simulink model "UIT"  (R2022b)
settings: Solver=VariableStepAuto  StartTime=0.0  StopTime=1e4  RelTol=1e-3
settings Model: Creator=lenovo  LastModifiedBy=lenovo

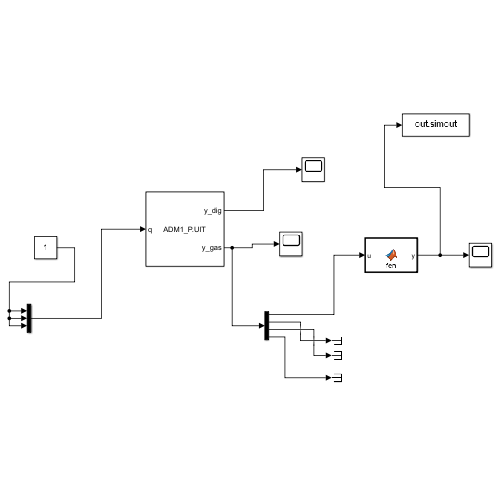
[thumbnail: Simulink's stored preview of the top-level diagram]
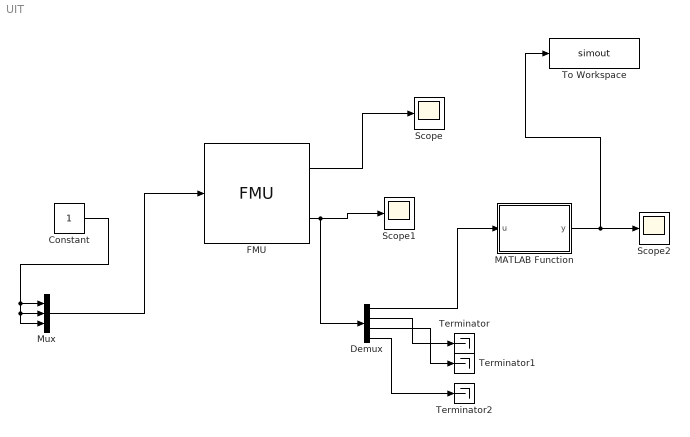
== system UIT ==
  Constant : Constant
  Demux : Demux
  FMU : FMU  FMUName=ADM1_P_UIT.fmu  FMUMode=ModelExchange  Gas_Meter=struct('D_ch4',1.57E-9,'D_co2',1.98E-9,'D_h2',4.65E-9,'D_n2',1.7777777777777777E-9,'D_nh3',1.9560185185185183E-9,'D_o2',2.8E-9,'P_atm',1.013,'T0',298.15,'T_op_mean',315.15,'T_ref_k',308.15,'V_gas',100.0,'V_liq',3400.0,'kla',200.0)  P_block_jacobian_check=off  P_block_jacobian_check_tol=1.0E-6  P_block_solver_experimental_mode=int32(0)  P_block_solver_profiling=off  P_cs_experimental_mode=int32(0)  P_cs_profiling=off  P_cs_rel_tol=1.0E-6  P_cs_solver=int32(0)  P_cs_step_size=0.001  P_enforce_bounds=on  P_events_default_tol=1.0E-10  P_events_tol_factor=1.0E-4  P_iteration_variable_scaling=int32(1)  P_log_level=int32(3)  P_log_start_time=-1.0E20  P_log_stop_time=1.0E20  P_mathematical_domain_warnings_limit=int32(-1)  P_nle_active_bounds_mode=int32(0)  P_nle_brent_ignore_error=off  P_nle_jacobian_calculation_mode=int32(0)  P_nle_jacobian_finite_difference_delta=1.490116119384766E-8  P_nle_jacobian_update_mode=int32(2)  P_nle_solver_check_jac_cond=off  P_nle_solver_default_tol=1.0E-10  P_nle_solver_exit_criterion=int32(3)  P_nle_solver_max_iter=int32(100)  P_nle_solver_max_iter_no_jacobian=int32(10)  P_nle_solver_max_residual_scaling_factor=1.0E10  P_nle_solver_min_residual_scaling_factor=1.0E-10  P_nle_solver_min_tol=1.0E-12  P_nle_solver_regularization_tolerance=-1.0  P_nle_solver_step_limit_factor=10.0  P_nle_solver_tol_factor=1.0E-4  P_nle_solver_use_last_integrator_step=on  P_nle_solver_use_nominals_as_fallback=on  P_rescale_after_singular_jac=on  P_rescale_each_step=off  P_residual_equation_scaling=int32(1)  P_runtime_log_to_file=off  P_time_events_default_tol=2.220446049250313E-14  P_use_Brent_in_1d=on  P_use_jacobian_equilibration=off  P_use_newton_for_brent=on  combiTimeTable=struct('columns',[int32(2),int32(3),int32(4),int32(5),int32(6),int32(7),int32(8),int32(9),int32(10),int32(11),int32(12),int32(13),int32(14),int32(15),int32(16),int32(17),int32(18),int32(19),int32(20),int32(21),int32(22),int32(23),int32(24),int32(25),int32(26),int32(27)],'offset',[0.0],'startTime',0.0,'table',reshape([0.0,1.0,2.0,0.0,1.0,4.0], [3,2]),'timeEvents',int32(1),'verboseRead',boolean(true))  combiTimeTable_fileName=C:/Users/lenovo/Desktop/KINGSTON/DOTTORATO/Modelica/Pilot_plant/Codig_Ari_Aprile 2023/txt_new/sAntonio_CattleSlurry_nir.txt  combiTimeTable_tableName=Input_CattleSlurry  combiTimeTable1=struct('columns',[int32(2),int32(3),int32(4),int32(5),int32(6),int32(7),int32(8),int32(9),int32(10),int32(11),int32(12),int32(13),int32(14),int32(15),int32(16),int32(17),int32(18),int32(19),int32(20),int32(21),int32(22),int32(23),int32(24),int32(25),int32(26),int32(27)],'offset',[0.0],'startTime',0.0,'table',reshape([0.0,1.0,2.0,0.0,1.0,4.0], [3,2]),'timeEvents',int32(1),'verboseRead',boolean(true))  combiTimeTable1_fileName=C:/Users/lenovo/Desktop/KINGSTON/DOTTORATO/Modelica/Pilot_plant/Codig_Ari_Aprile 2023/txt_new/sAntonio_MaizeSilage_nir.txt  combiTimeTable1_tableName=Input_MaizeSilage  combiTimeTable2=struct('columns',[int32(2),int32(3),int32(4),int32(5),int32(6),int32(7),int32(8),int32(9),int32(10),int32(11),int32(12),int32(13),int32(14),int32(15),int32(16),int32(17),int32(18),int32(19),int32(20),int32(21),int32(22),int32(23),int32(24),int32(25),int32(26),int32(27)],'offset',[0.0],'startTime',0.0,'table',reshape([0.0,1.0,2.0,0.0,1.0,4.0], [3,2]),'timeEvents',int32(1),'verboseRead',boolean(true))  combiTimeTable2_fileName=C:/Users/lenovo/Desktop/KINGSTON/DOTTORATO/Modelica/Pilot_plant/Codig_Ari_Aprile 2023/txt_new/UIT_TomatoSouce_nir.txt  combiTimeTable2_tableName=Input_TomatoSouce  combiTimeTable3=struct('columns',[int32(2),int32(3),int32(4),int32(5),int32(6),int32(7),int32(8),int32(9),int32(10),int32(11),int32(12),int32(13),int32(14),int32(15),int32(16),int32(17),int32(18),int32(19),int32(20),int32(21),int32(22),int32(23),int32(24),int32(25),int32(26),int32(27)],'offset',[0.0],'startTime',0.0,'table',reshape([0.0,1.0,2.0,0.0,1.0,4.0], [3,2]),'timeEvents',int32(1),'verboseRead',boolean(true))  combiTimeTable3_fileName=C:/Users/lenovo/Desktop/KINGSTON/DOTTORATO/Modelica/Pilot_plant/Codig_Ari_Aprile 2023/txt_new/sAntonio_TomatoPeels_nir.txt  combiTimeTable3_tableName=Input_TomatoPeels  combiTimeTable4=struct('columns',[int32(2)],'offset',[0.0],'startTime',0.0,'table',reshape([0.0,150.0,240.0,2000.0,0.0,37.0,0.0,37.0], [4,2]),'timeEvents',int32(1),'verboseRead',boolean(true))  combiTimeTable4_fileName=NoName  combiTimeTable4_tableName=NoName  combiTimeTable5=struct('columns',[int32(2)],'offset',[0.0],'startTime',0.0,'table',reshape([0.0,150.0,240.0,2000.0,37.0,0.0,37.0,37.0], [4,2]),'timeEvents',int32(1),'verboseRead',boolean(true))  combiTimeTable5_fileName=NoName  combiTimeTable5_tableName=NoName  digester=struct('COD_VS_PR_BCA',1.58,'D_ch4',1.57E-9,'D_co2',1.98E-9,'D_h2',4.65E-9,'D_n2',1.7777777777777777E-9,'D_nh3',1.9560185185185183E-9,'D_o2',2.8E-9,'Ki_h2_c4',1.0E-5,'Ki_h2_fa',5.0E-6,'Ki_h2_pro',3.5E-6,'Ki_nh3_ac',0.0018,'Ks_IN',1.0E-4,'Ks_IP',2.0E-5,'Ks_aa',0.3,'Ks_ac',0.15,'Ks_c4',0.1,'Ks_fa',0.4,'Ks_h2',2.5E-5,'Ks_pro',0.3,'Ks_su',0.5,'N_PR',7.5,'P_atm',1.013,'S_aa_start',0.0260061,'S_ac_start',0.259353,'S_an_start',0.0156,'S_bu_start',0.00643617,'S_ca_start',3.28398E-5,'S_cat_start',0.121528,'S_ch4_start',0.277401,'S_fa_start',0.0444521,'S_gas_ch4_start',1.27265,'S_gas_co2_start',0.0164995,'S_gas_h2_start',5.30538E-6,'S_gas_nh3_start',3.35695E-6,'S_h2_start',6.87765E-7,'S_i_start',0.193985,'S_ic_start',0.255202,'S_in_start',0.157029,'S_ip_start',0.00496694,'S_mg_start',5.62229E-5,'S_pro_start',0.050891,'S_su_start',0.0246664,'S_va_start',0.00353521,'T0',298.15,'T_op_mean',315.15,'T_ref',298.15,'T_ref_k',308.15,'Tref_khyd',[308.15,308.15,308.15,308.15,308.15,308.15,308.15,308.15],'V_gas',0.0172,'V_liq',0.012,'X_aa_start',0.566877,'X_ac_start',1.32145,'X_acp_start',8.78817E-12,'X_c4_start',0.498118,'X_c_start',0.0,'X_ccm_start',0.00543116,'X_ch_start',[0.82044,0.712461,10.3487],'X_fa_start',0.288931,'X_h2_start',0.621273,'X_i_start',36.0924,'X_li_start',0.707873,'X_lig_start',13.3149,'X_mag_start',1.41797E-9,'X_p_start',0.77594,'X_pr_start',[0.140817,0.868087],'X_pro_start',0.316025,'X_stru_start',0.0100858,'X_su_start',2.61837,'Y_aa',0.08,'Y_ac',0.05,'Y_c4',0.06,'Y_fa',0.06,'Y_h2',0.06,'Y_pro',0.04,'Y_su',0.1,'ash_start',14.1091,'convKa',1.0,'f_ac_aa',0.4,'f_bu_aa',0.26,'f_ch_xb',0.275,'f_fa_li',0.95,'f_h2_aa',0.06,'f_li_xb',0.35,'f_pr_xb',0.275,'f_pro_aa',0.05,'f_si_xb',0.02,'f_va_aa',0.23,'f_xi_xb',0.08,'ideality',boolean(false),'k_dec_aa',0.02,'k_dec_ac',0.02,'k_dec_c4',0.02,'k_dec_fa',0.02,'k_dec_h2',0.02,'k_dec_pro',0.02,'k_dec_su',0.02,'k_dis',1.2,'k_hyd_xchm',0.3,'k_hyd_xchr',1.0,'k_hyd_xchs',0.01,'k_hyd_xcr',0.1,'k_hyd_xcs',0.01,'k_hyd_xli',0.3,'k_hyd_xprr',1.0,'k_hyd_xprs',0.2,'k_m_aa',8.0,'k_m_ac',5.6,'k_m_c4',14.0,'k_m_fa',8.0,'k_m_h2',35.0,'k_m_pro',13.0,'k_m_su',11.0,'kla',10.0,'multihyd',boolean(true),'nW',int32(1),'noXc',boolean(true),'nu_1_su',0.495,'nu_2_su',0.345,'pH_LL_aa',4.0,'pH_LL_ac',6.0,'pH_LL_h2',5.0,'pH_UL_aa',5.5,'pH_UL_ac',7.0,'pH_UL_h2',6.0,'precipitation',boolean(true))  limPID=struct('Dzero',struct('k',0.0),'FFzero',struct('k',0.0),'Nd',10.0,'Ni',0.9,'P',struct('k',1.0),'Td',0.1,'Ti',43200.0,'addFF',struct('k1',1.0),'addI',struct('k1',1.0,'k2',-1.0,'k3',1.0),'addP',struct('k2',-1.0),'addPID',struct('k1',1.0,'k2',1.0,'k3',1.0),'addSat',struct('k1',1.0,'k2',-1.0),'k',0.73,'kFF',1.0,'wd',0.0,'wp',1.0,'xd_start',0.0,'xi_start',0.0235182)  maize=struct('COD_VS_PR_BCA',1.58,'N_PR',7.5,'T_ref',298.15,'Y_aa',0.08,'Y_ac',0.05,'Y_c4',0.06,'Y_fa',0.06,'Y_h2',0.06,'Y_pro',0.04,'Y_su',0.1,'aa',0.0,'ac',0.0,'adl',0.0,'an',0.0,'bd_cell',50.0,'bd_hemicell',50.0,'bd_li',50.0,'bd_pr',50.0,'bu',0.0,'ca',0.0,'cat',0.0,'cellulose',0.0,'ch4',0.0,'convKa',1.0,'f_Xbiom_ch',0.195,'f_Xbiom_pr',0.8,'f_ac_aa',0.4,'f_bu_aa',0.26,'f_ch_xb',0.275,'f_fa_li',0.95,'f_h2_aa',0.06,'f_li_xb',0.35,'f_pr_r',0.5,'f_pr_s',0.5,'f_pr_xb',0.275,'f_pro_aa',0.05,'f_si_xb',0.02,'f_va_aa',0.23,'f_xi_xb',0.08,'fa',0.0,'h2',0.0,'hemicellulose',0.0,'lipid',0.0,'liquid',boolean(false),'mg',0.0,'nu_1_su',0.495,'nu_2_su',0.345,'ortop',0.0,'ph',0.0,'pro',0.0,'protein',0.0,'si',0.0,'starch',0.0,'steady',boolean(false),'su',0.0,'tac',0.0,'tan',764.0,'tbmp_vs',0.0,'tic',0.0,'ts',0.0,'va',0.0,'vs_ts',0.0,'xaa',0.0,'xac',0.0,'xc4',0.0,'xfa',0.0,'xh2',0.0,'xpro',0.0,'xsu',0.0)  nW=int32(1)  nXin=int32(30)  sampler_with_oclk=struct('Ts_2',500000.0)  sampler_with_oclk1=struct('Ts_2',500000.0)  sink_vec=struct('COD_VS_PR_BCA',1.58,'N_PR',7.5,'Y_aa',0.08,'Y_ac',0.05,'Y_c4',0.06,'Y_fa',0.06,'Y_h2',0.06,'Y_pro',0.04,'Y_su',0.1,'f_Xbiom_ch',0.195,'f_Xbiom_pr',0.8,'f_ac_aa',0.4,'f_bu_aa',0.26,'f_ch_si',0.6,'f_ch_xb',0.275,'f_ch_xc',0.2,'f_ch_xi',0.1,'f_fa_li',0.95,'f_h2_aa',0.06,'f_li_xb',0.35,'f_li_xc',0.2,'f_lig_xc',0.1,'f_pr_si',0.4,'f_pr_xb',0.275,'f_pr_xc',0.2,'f_pr_xi',0.55,'f_pro_aa',0.05,'f_si_xb',0.02,'f_va_aa',0.23,'f_xi_xb',0.08,'f_xi_xc',0.2,'nu_1_su',0.495,'nu_2_su',0.345)  sink_vec1=struct('COD_VS_PR_BCA',1.58,'N_PR',7.5,'Y_aa',0.08,'Y_ac',0.05,'Y_c4',0.06,'Y_fa',0.06,'Y_h2',0.06,'Y_pro',0.04,'Y_su',0.1,'f_Xbiom_ch',0.195,'f_Xbiom_pr',0.8,'f_ac_aa',0.4,'f_bu_aa',0.26,'f_ch_si',0.6,'f_ch_xb',0.275,'f_ch_xc',0.2,'f_ch_xi',0.1,'f_fa_li',0.95,'f_h2_aa',0.06,'f_li_xb',0.35,'f_li_xc',0.2,'f_lig_xc',0.1,'f_pr_si',0.4,'f_pr_xb',0.275,'f_pr_xc',0.2,'f_pr_xi',0.55,'f_pro_aa',0.05,'f_si_xb',0.02,'f_va_aa',0.23,'f_xi_xb',0.08,'f_xi_xc',0.2,'nu_1_su',0.495,'nu_2_su',0.345)  slurry=struct('COD_VS_PR_BCA',1.58,'N_PR',7.5,'T_ref',298.15,'Y_aa',0.08,'Y_ac',0.05,'Y_c4',0.06,'Y_fa',0.06,'Y_h2',0.06,'Y_pro',0.04,'Y_su',0.1,'aa',0.0,'ac',0.0,'adl',0.0,'an',0.02,'bd_cell',50.0,'bd_hemicell',50.0,'bd_li',50.0,'bd_pr',50.0,'bu',0.0,'ca',0.0,'cat',0.0,'cellulose',0.0,'ch4',0.0,'convKa',1.0,'f_Xbiom_ch',0.195,'f_Xbiom_pr',0.8,'f_ac_aa',0.4,'f_bu_aa',0.26,'f_ch_xb',0.275,'f_fa_li',0.95,'f_h2_aa',0.06,'f_li_xb',0.35,'f_pr_r',0.5,'f_pr_s',0.5,'f_pr_xb',0.275,'f_pro_aa',0.05,'f_si_xb',0.02,'f_va_aa',0.23,'f_xi_xb',0.08,'fa',0.0,'h2',0.0,'hemicellulose',0.0,'lipid',0.0,'liquid',boolean(true),'mg',0.0,'nu_1_su',0.495,'nu_2_su',0.345,'ortop',0.0,'ph',0.0,'pro',0.0,'protein',0.0,'si',0.0,'starch',0.0,'steady',boolean(false),'su',0.0,'tac',0.0,'tan',0.0,'tbmp_vs',0.0,'tic',0.0,'ts',0.0,'va',0.0,'vs_ts',0.0,'xaa',0.0,'xac',0.0,'xc4',0.0,'xfa',0.0,'xh2',0.0,'xpro',0.0,'xsu',0.0)  step=struct('height',0.0,'offset',1.035,'startTime',1000000.0)  timeTable=struct('offset',0.0,'startTime',0.0,'table',reshape([0.0,2000.0,315.15,315.15], [2,2]))  timeTable1=struct('offset',0.0,'startTime',0.0,'table',reshape([0.0,2000.0,315.15,315.15], [2,2]))  tomatopeels=struct('COD_VS_PR_BCA',1.58,'N_PR',7.5,'T_ref',298.15,'Y_aa',0.08,'Y_ac',0.05,'Y_c4',0.06,'Y_fa',0.06,'Y_h2',0.06,'Y_pro',0.04,'Y_su',0.1,'aa',0.0,'ac',0.0,'adl',0.0,'an',0.0,'bd_cell',50.0,'bd_hemicell',50.0,'bd_li',50.0,'bd_pr',50.0,'bu',0.0,'ca',0.0,'cat',0.0,'cellulose',0.0,'ch4',0.0,'convKa',1.0,'f_Xbiom_ch',0.195,'f_Xbiom_pr',0.8,'f_ac_aa',0.4,'f_bu_aa',0.26,'f_ch_xb',0.275,'f_fa_li',0.95,'f_h2_aa',0.06,'f_li_xb',0.35,'f_pr_r',0.5,'f_pr_s',0.5,'f_pr_xb',0.275,'f_pro_aa',0.05,'f_si_xb',0.02,'f_va_aa',0.23,'f_xi_xb',0.08,'fa',0.0,'h2',0.0,'hemicellulose',0.0,'lipid',0.0,'liquid',boolean(false),'mg',0.0,'nW',int32(1),'nXin',int32(26),'nu_1_su',0.495,'nu_2_su',0.345,'ortop',0.0,'ph',0.0,'pro',0.0,'protein',0.0,'si',0.0,'starch',0.0,'steady',boolean(false),'su',0.0,'tac',0.0,'tan',764.0,'tbmp_vs',0.0,'tic',0.0,'ts',0.0,'va',0.0,'vs_ts',0.0,'xaa',0.0,'xac',0.0,'xc4',0.0,'xfa',0.0,'xh2',0.0,'xpro',0.0,'xsu',0.0)  tomatosouce=struct('COD_VS_PR_BCA',1.58,'N_PR',7.5,'T_ref',298.15,'Y_aa',0.08,'Y_ac',0.05,'Y_c4',0.06,'Y_fa',0.06,'Y_h2',0.06,'Y_pro',0.04,'Y_su',0.1,'aa',0.0,'ac',0.0,'adl',0.0,'an',0.02,'bd_cell',50.0,'bd_hemicell',50.0,'bd_li',50.0,'bd_pr',50.0,'bu',0.0,'ca',0.0,'cat',0.0,'cellulose',0.0,'ch4',0.0,'convKa',1.0,'f_Xbiom_ch',0.195,'f_Xbiom_pr',0.8,'f_ac_aa',0.4,'f_bu_aa',0.26,'f_ch_xb',0.275,'f_fa_li',0.95,'f_h2_aa',0.06,'f_li_xb',0.35,'f_pr_r',1.0,'f_pr_s',0.0,'f_pr_xb',0.275,'f_pro_aa',0.05,'f_si_xb',0.02,'f_va_aa',0.23,'f_xi_xb',0.08,'fa',0.0,'h2',0.0,'hemicellulose',0.0,'lipid',0.0,'liquid',boolean(true),'mg',0.0,'nu_1_su',0.495,'nu_2_su',0.345,'ortop',0.0,'ph',0.0,'pro',0.0,'protein',0.0,'si',0.0,'starch',0.0,'steady',boolean(false),'su',0.0,'tac',0.0,'tan',0.0,'tbmp_vs',0.0,'tic',0.0,'ts',0.0,'va',0.0,'vs_ts',0.0,'xaa',0.0,'xac',0.0,'xc4',0.0,'xfa',0.0,'xh2',0.0,'xpro',0.0,'xsu',0.0)  mask(ADM1_P.UIT [Model Exchange, v2.0]){}
      settings: MultithreadedSim=off
      mask Display:
      | disp('ADM1_P.UIT');
      | port_label('output',1,'y_dig');
      | port_label('output',2,'y_gas');
      | port_label('input',1,'q');
  MATLAB Function : MATLAB Function  TreatAsAtomicUnit=on
  Mux : Mux  Inputs=3
  Scope : Scope
  Scope1 : Scope
  Scope2 : Scope
  Terminator : Terminator
  Terminator1 : Terminator
  Terminator2 : Terminator
  To Workspace : ToWorkspace  VariableName=simout  SaveFormat=Timeseries  SampleTime=-1
  wires:
  Mux/1 -> FMU/1
  Constant/1 -> Mux/3, Mux/2, Mux/1
  FMU/1 -> Scope/1
  FMU/2 -> Demux/1, Scope1/1
  MATLAB Function/1(y) -> To Workspace/1, Scope2/1
  Demux/1 -> MATLAB Function/1(u)
  Demux/2 -> Terminator/1
  Demux/3 -> Terminator1/1
  Demux/4 -> Terminator2/1

== matlab function UIT/MATLAB Function ==
  data: u input; y output
function y = fcn(u)
T = 1e4;
measurment = [1 3;10 20;30 50];
t_meas = measurment(:,1);
meas = measurment(:,2);
i_curr = 1;
err = zeros(T,1);
y_cum=zeros(T,1);
for i = 1:T
    if (i_curr <= size(t_meas,1) && i==t_meas(i_curr) )
        err(i) = u(i) - meas(i_curr);
        i_curr = i_curr+1;
    end
end
y = sum(err)
